simulink subsystem "gimbal_control_sub"  (R2025b)
settings: Solver=VariableStepAuto  StartTime=0.0  StopTime=10.0  RelTol=1e-3
libraries: simulink_extras x2
settings Model: Creator=lew11  LastModifiedBy=lew11

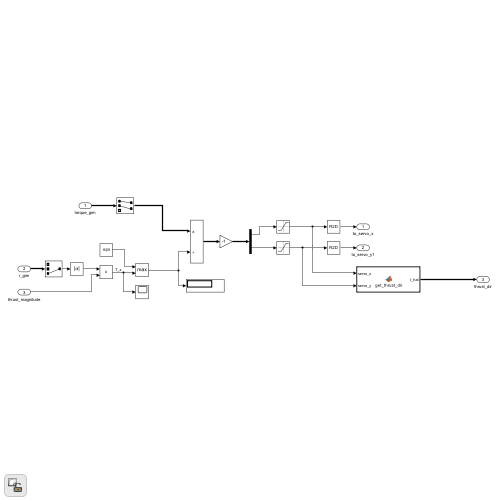
[thumbnail: Simulink's stored preview of the top-level diagram]
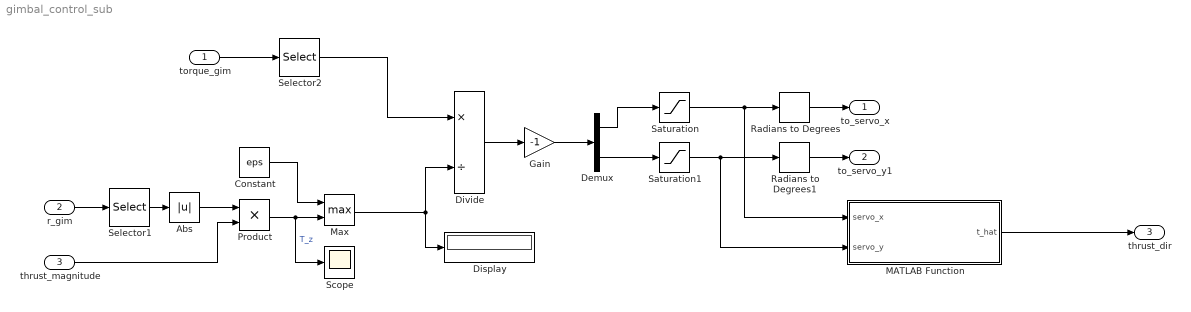
== system gimbal_control_sub ==
  torque_gim : Inport  PortDimensions=3
  r_gim : Inport  Port=2  PortDimensions=3
  thrust_magnitude : Inport  Port=3  Unit=N  PortDimensions=1
  Abs : Abs  SaturateOnIntegerOverflow=off
  Constant : Constant  Value=eps
  Demux : Demux  Outputs=2
  Display : Display
  Divide : Product  Inputs=*/
  Gain : Gain  Gain=-1
  MATLAB Function : MATLAB Function  TreatAsAtomicUnit=on
  Max : MinMax  Function=max  Inputs=2
  Product : Product
  Radians to Degrees : simulink_extras/Transformations/Radians to Degrees
  Radians to Degrees1 : simulink_extras/Transformations/Radians to Degrees
  Saturation : Saturate  UpperLimit=deg2rad(15)  LowerLimit=deg2rad(-15)
  Saturation1 : Saturate  UpperLimit=deg2rad(15)  LowerLimit=deg2rad(-15)
  Scope : Scope
      settings: ActiveDisplayYMinimum=3.0167440358180659  ActiveDisplayYMaximum=9.5381628970097587  DataLoggingVariableName=ScopeData13
  Selector1 : Selector  InputPortWidth=3  IndexOptions=Index vector (dialog)  Indices=[3]  OutputSizes=1
  Selector2 : Selector  InputPortWidth=3  IndexOptions=Index vector (dialog)  Indices=[1 2]  OutputSizes=1
  to_servo_x : Outport  PortDimensions=1
  to_servo_y1 : Outport  Port=2  PortDimensions=1
  thrust_dir : Outport  Port=3
  wires:
  Saturation1/1 -> MATLAB Function/2(servo_y), Radians to Degrees1/1
  Radians to Degrees1/1 -> to_servo_y1/1
  Abs/1 -> Product/1
  Selector2/1 -> Divide/1
  Demux/1 -> Saturation/1
  Divide/1 -> Gain/1
  thrust_magnitude/1 -> Product/2
  torque_gim/1 -> Selector2/1
  Selector1/1 -> Abs/1
  MATLAB Function/1(t_hat) -> thrust_dir/1
  r_gim/1 -> Selector1/1
  Saturation/1 -> MATLAB Function/1(servo_x), Radians to Degrees/1
  Demux/2 -> Saturation1/1
  Radians to Degrees/1 -> to_servo_x/1
  Product/1 -> Max/2, Scope/1  "T_z"
  Constant/1 -> Max/1
  Max/1 -> Display/1, Divide/2
  Gain/1 -> Demux/1

== matlab function gimbal_control_sub/MATLAB Function ==
  data: servo_x input; t_hat output; servo_y input
function t_hat = get_thrust_dir(servo_x, servo_y)

t_x = -servo_y;
t_y = servo_x;
t_z = -1 + (servo_x^2+servo_y^2)/2;

t_hat = [t_x; t_y; t_z];
